simulink model "DiskBrakeThermal"  (R2025b)
settings: Solver=ode45  StartTime=0.0  StopTime=520  MaxStep=0.1  RelTol=1e-6
PreLoadFcn:
  | disk_brake_thermal_params
values from neighbouring files (symbols this model uses):
  A_backing = 0.004    [disk_brake_thermal_params.m]
  A_contact = 0.004    [disk_brake_thermal_params.m]
  A_piston = 0.0012    [disk_brake_thermal_params.m]
  A_rotor = 0.12    [disk_brake_thermal_params.m]
  c_b = 490    [disk_brake_thermal_params.m]
  c_p = 935    [disk_brake_thermal_params.m]
  c_r = 449    [disk_brake_thermal_params.m]
  Cd_A = 0.72    [disk_brake_thermal_params.m]
  Cr = 0.012    [disk_brake_thermal_params.m]
  D = 0.28    [disk_brake_thermal_params.m]
  eps_r = 0.40    (= 0.4)    [disk_brake_thermal_params.m]
  F_drive_max = 7000    [disk_brake_thermal_params.m]
  g = 9.81    [disk_brake_thermal_params.m]
  gamma = 0.95    [disk_brake_thermal_params.m]
  h_nat = 8    [disk_brake_thermal_params.m]
  k_air = 0.026    [disk_brake_thermal_params.m]
  k_cond_pb = k_b * A_backing / t_b    (= 36)    [disk_brake_thermal_params.m]
  k_cond_rp = k_p * A_contact / t_pad    (= 2.9)    [disk_brake_thermal_params.m]
  m_b = 0.25    [disk_brake_thermal_params.m]
  m_p = 0.30    (= 0.3)    [disk_brake_thermal_params.m]
  m_r = 6.0    (= 6)    [disk_brake_thermal_params.m]
  m_veh = 1700    [disk_brake_thermal_params.m]
  mu_air = 1.8e-5    (= 1.8e-05)    [disk_brake_thermal_params.m]
  mu_pad = 0.40    (= 0.4)    [disk_brake_thermal_params.m]
  P_line_max = 120e5    (= 12000000)    [disk_brake_thermal_params.m]
  R_eff = 0.11    [disk_brake_thermal_params.m]
  R_wheel = 0.32    [disk_brake_thermal_params.m]
  rho_air = 1.17    [disk_brake_thermal_params.m]
  rho_air_drag = 1.225    [disk_brake_thermal_params.m]
  sigma = 5.67e-8    (= 5.67e-08)    [disk_brake_thermal_params.m]
  T_amb_init = 25    [disk_brake_thermal_params.m]
  v0 = 27.8    [disk_brake_thermal_params.m]
settings Model: Creator=grouleau  LastModifiedBy=grouleau
settings DataIOCC: ExternalInput=ext_input  LoadExternalInput=on

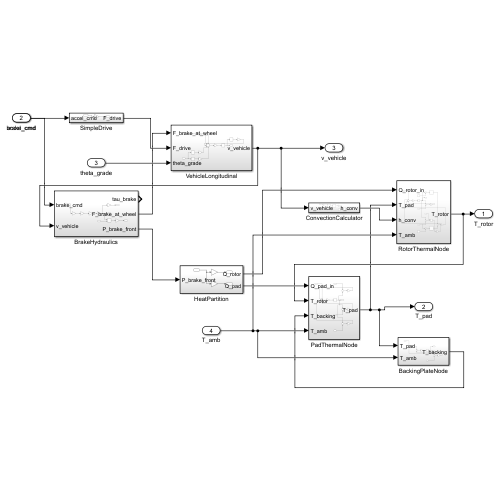
[thumbnail: Simulink's stored preview of the top-level diagram]
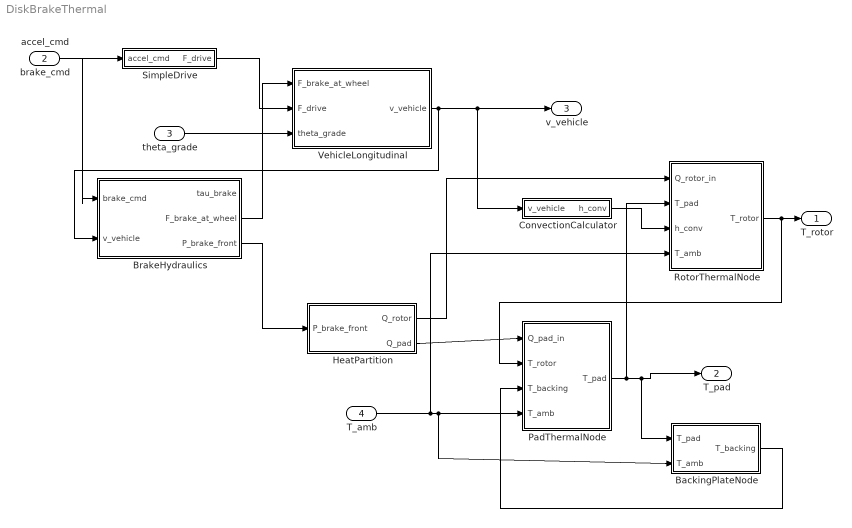
== system DiskBrakeThermal ==
  brake_cmd : Inport
  accel_cmd : Inport  Port=2
  theta_grade : Inport  Port=3
  T_amb : Inport  Port=4
  BackingPlateNode : Subsystem
  BrakeHydraulics : Subsystem
  ConvectionCalculator : Subsystem
  HeatPartition : Subsystem
  PadThermalNode : Subsystem
  RotorThermalNode : Subsystem
  SimpleDrive : Subsystem
  VehicleLongitudinal : Subsystem
  T_rotor : Outport
  T_pad : Outport  Port=2
  v_vehicle : Outport  Port=3
  wires:
  brake_cmd/1 -> BrakeHydraulics/1(brake_cmd)
  accel_cmd/1 -> SimpleDrive/1(accel_cmd)
  theta_grade/1 -> VehicleLongitudinal/3(theta_grade)
  BrakeHydraulics/2(F_brake_at_wheel) -> VehicleLongitudinal/1(F_brake_at_wheel)
  SimpleDrive/1(F_drive) -> VehicleLongitudinal/2(F_drive)
  VehicleLongitudinal/1(v_vehicle) -> v_vehicle/1, ConvectionCalculator/1(v_vehicle), BrakeHydraulics/2(v_vehicle)
  BrakeHydraulics/3(P_brake_front) -> HeatPartition/1(P_brake_front)
  HeatPartition/1(Q_rotor) -> RotorThermalNode/1(Q_rotor_in)
  HeatPartition/2(Q_pad) -> PadThermalNode/1(Q_pad_in)
  ConvectionCalculator/1(h_conv) -> RotorThermalNode/3(h_conv)
  T_amb/1 -> BackingPlateNode/2(T_amb), PadThermalNode/4(T_amb), RotorThermalNode/4(T_amb)
  RotorThermalNode/1(T_rotor) -> PadThermalNode/2(T_rotor), T_rotor/1
  PadThermalNode/1(T_pad) -> T_pad/1, BackingPlateNode/1(T_pad), RotorThermalNode/2(T_pad)
  BackingPlateNode/1(T_backing) -> PadThermalNode/3(T_backing)

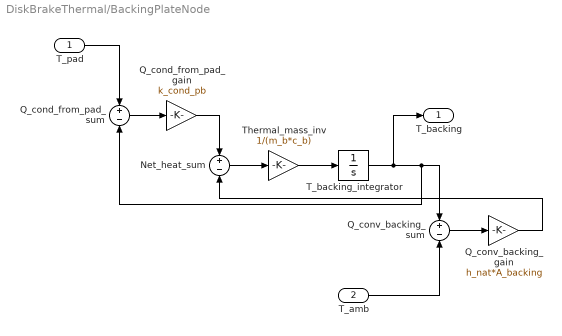
== system DiskBrakeThermal/BackingPlateNode ==
  T_pad : Inport
  T_amb : Inport  Port=2
  Net_heat_sum : Sum  Inputs=+-
  Q_cond_from_pad_gain : Gain  Gain=k_cond_pb
  Q_cond_from_pad_sum : Sum  Inputs=+-
  Q_conv_backing_gain : Gain  Gain=h_nat*A_backing
  Q_conv_backing_sum : Sum  Inputs=+-
  T_backing_integrator : Integrator  InitialCondition=T_amb_init
  Thermal_mass_inv : Gain  Gain=1/(m_b*c_b)
  T_backing : Outport
  wires:
  T_pad/1 -> Q_cond_from_pad_sum/1
  Q_cond_from_pad_sum/1 -> Q_cond_from_pad_gain/1
  Q_conv_backing_sum/1 -> Q_conv_backing_gain/1
  Q_cond_from_pad_gain/1 -> Net_heat_sum/1
  Q_conv_backing_gain/1 -> Net_heat_sum/2
  Net_heat_sum/1 -> Thermal_mass_inv/1
  Thermal_mass_inv/1 -> T_backing_integrator/1
  T_backing_integrator/1 -> Q_conv_backing_sum/1, Q_cond_from_pad_sum/2, T_backing/1
  T_amb/1 -> Q_conv_backing_sum/2

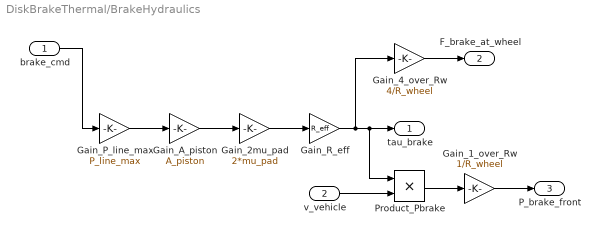
== system DiskBrakeThermal/BrakeHydraulics ==
  brake_cmd : Inport
  v_vehicle : Inport  Port=2
  Gain_1_over_Rw : Gain  Gain=1/R_wheel
  Gain_2mu_pad : Gain  Gain=2*mu_pad
  Gain_4_over_Rw : Gain  Gain=4/R_wheel
  Gain_A_piston : Gain  Gain=A_piston
  Gain_P_line_max : Gain  Gain=P_line_max
  Gain_R_eff : Gain  Gain=R_eff
  Product_Pbrake : Product
  tau_brake : Outport
  F_brake_at_wheel : Outport  Port=2
  P_brake_front : Outport  Port=3
  wires:
  brake_cmd/1 -> Gain_P_line_max/1
  Gain_P_line_max/1 -> Gain_A_piston/1
  Gain_A_piston/1 -> Gain_2mu_pad/1
  Gain_2mu_pad/1 -> Gain_R_eff/1
  Gain_R_eff/1 -> Product_Pbrake/1, tau_brake/1, Gain_4_over_Rw/1
  Gain_4_over_Rw/1 -> F_brake_at_wheel/1
  v_vehicle/1 -> Product_Pbrake/2
  Product_Pbrake/1 -> Gain_1_over_Rw/1
  Gain_1_over_Rw/1 -> P_brake_front/1

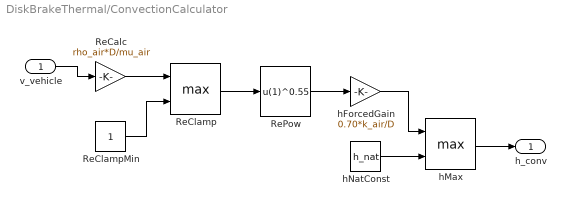
== system DiskBrakeThermal/ConvectionCalculator ==
  v_vehicle : Inport
  ReCalc : Gain  Gain=rho_air*D/mu_air
  ReClamp : MinMax  Function=max  Inputs=2
  ReClampMin : Constant
  RePow : Fcn  Expr=u(1)^0.55
  hForcedGain : Gain  Gain=0.70*k_air/D
  hMax : MinMax  Function=max  Inputs=2
  hNatConst : Constant  Value=h_nat
  h_conv : Outport
  wires:
  v_vehicle/1 -> ReCalc/1
  ReCalc/1 -> ReClamp/1
  ReClampMin/1 -> ReClamp/2
  ReClamp/1 -> RePow/1
  RePow/1 -> hForcedGain/1
  hForcedGain/1 -> hMax/1
  hNatConst/1 -> hMax/2
  hMax/1 -> h_conv/1

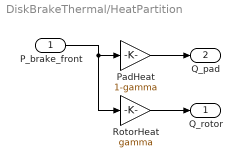
== system DiskBrakeThermal/HeatPartition ==
  P_brake_front : Inport
  PadHeat : Gain  Gain=1-gamma
  RotorHeat : Gain  Gain=gamma
  Q_rotor : Outport
  Q_pad : Outport  Port=2
  wires:
  P_brake_front/1 -> PadHeat/1, RotorHeat/1
  RotorHeat/1 -> Q_rotor/1
  PadHeat/1 -> Q_pad/1

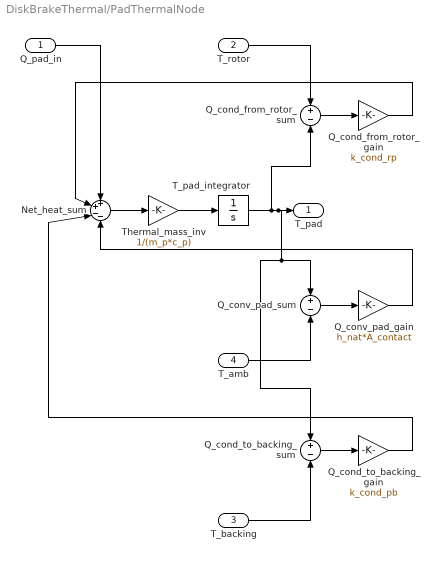
== system DiskBrakeThermal/PadThermalNode ==
  Q_pad_in : Inport
  T_rotor : Inport  Port=2
  T_backing : Inport  Port=3
  T_amb : Inport  Port=4
  Net_heat_sum : Sum  Inputs=++--
  Q_cond_from_rotor_gain : Gain  Gain=k_cond_rp
  Q_cond_from_rotor_sum : Sum  Inputs=+-
  Q_cond_to_backing_gain : Gain  Gain=k_cond_pb
  Q_cond_to_backing_sum : Sum  Inputs=+-
  Q_conv_pad_gain : Gain  Gain=h_nat*A_contact
  Q_conv_pad_sum : Sum  Inputs=+-
  T_pad_integrator : Integrator  InitialCondition=T_amb_init
  Thermal_mass_inv : Gain  Gain=1/(m_p*c_p)
  T_pad : Outport
  wires:
  T_rotor/1 -> Q_cond_from_rotor_sum/1
  Q_cond_from_rotor_sum/1 -> Q_cond_from_rotor_gain/1
  Q_cond_to_backing_sum/1 -> Q_cond_to_backing_gain/1
  Q_conv_pad_sum/1 -> Q_conv_pad_gain/1
  Q_pad_in/1 -> Net_heat_sum/1
  Q_cond_from_rotor_gain/1 -> Net_heat_sum/2
  Q_cond_to_backing_gain/1 -> Net_heat_sum/3
  Q_conv_pad_gain/1 -> Net_heat_sum/4
  Net_heat_sum/1 -> Thermal_mass_inv/1
  Thermal_mass_inv/1 -> T_pad_integrator/1
  T_pad_integrator/1 -> Q_conv_pad_sum/1, Q_cond_to_backing_sum/1, T_pad/1, Q_cond_from_rotor_sum/2
  T_backing/1 -> Q_cond_to_backing_sum/2
  T_amb/1 -> Q_conv_pad_sum/2

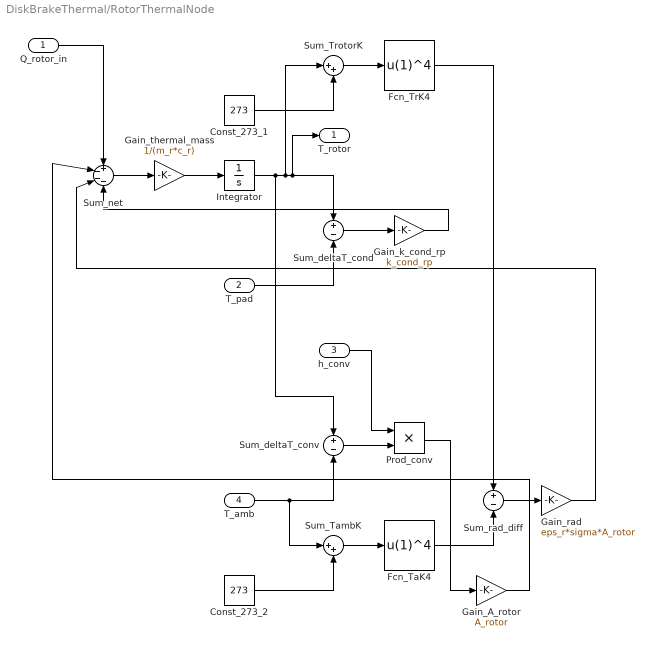
== system DiskBrakeThermal/RotorThermalNode ==
  Q_rotor_in : Inport
  T_pad : Inport  Port=2
  h_conv : Inport  Port=3
  T_amb : Inport  Port=4
  Const_273_1 : Constant  Value=273
  Const_273_2 : Constant  Value=273
  Fcn_TaK4 : Fcn  Expr=u(1)^4
  Fcn_TrK4 : Fcn  Expr=u(1)^4
  Gain_A_rotor : Gain  Gain=A_rotor
  Gain_k_cond_rp : Gain  Gain=k_cond_rp
  Gain_rad : Gain  Gain=eps_r*sigma*A_rotor
  Gain_thermal_mass : Gain  Gain=1/(m_r*c_r)
  Integrator : Integrator  InitialCondition=T_amb_init
  Prod_conv : Product
  Sum_TambK : Sum  Inputs=|++
  Sum_TrotorK : Sum  Inputs=|++
  Sum_deltaT_cond : Sum  Inputs=+-
  Sum_deltaT_conv : Sum  Inputs=+-
  Sum_net : Sum  Inputs=+---
  Sum_rad_diff : Sum  Inputs=+-
  T_rotor : Outport
  wires:
  Integrator/1 -> T_rotor/1, Sum_deltaT_cond/1, Sum_TrotorK/1, Sum_deltaT_conv/1
  T_amb/1 -> Sum_TambK/1, Sum_deltaT_conv/2
  h_conv/1 -> Prod_conv/1
  Sum_deltaT_conv/1 -> Prod_conv/2
  Prod_conv/1 -> Gain_A_rotor/1
  Const_273_1/1 -> Sum_TrotorK/2
  Const_273_2/1 -> Sum_TambK/2
  Sum_TrotorK/1 -> Fcn_TrK4/1
  Sum_TambK/1 -> Fcn_TaK4/1
  Fcn_TrK4/1 -> Sum_rad_diff/1
  Fcn_TaK4/1 -> Sum_rad_diff/2
  Sum_rad_diff/1 -> Gain_rad/1
  T_pad/1 -> Sum_deltaT_cond/2
  Sum_deltaT_cond/1 -> Gain_k_cond_rp/1
  Sum_net/1 -> Gain_thermal_mass/1
  Gain_thermal_mass/1 -> Integrator/1
  Q_rotor_in/1 -> Sum_net/1
  Gain_A_rotor/1 -> Sum_net/2
  Gain_rad/1 -> Sum_net/3
  Gain_k_cond_rp/1 -> Sum_net/4

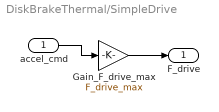
== system DiskBrakeThermal/SimpleDrive ==
  accel_cmd : Inport
  Gain_F_drive_max : Gain  Gain=F_drive_max
  F_drive : Outport
  wires:
  accel_cmd/1 -> Gain_F_drive_max/1
  Gain_F_drive_max/1 -> F_drive/1

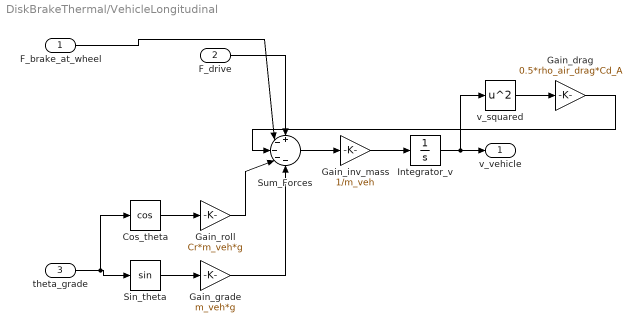
== system DiskBrakeThermal/VehicleLongitudinal ==
  F_brake_at_wheel : Inport
  F_drive : Inport  Port=2
  theta_grade : Inport  Port=3
  Cos_theta : Trigonometry  Operator=cos  ApproximationMethod=CORDIC
  Gain_drag : Gain  Gain=0.5*rho_air_drag*Cd_A
  Gain_grade : Gain  Gain=m_veh*g
  Gain_inv_mass : Gain  Gain=1/m_veh
  Gain_roll : Gain  Gain=Cr*m_veh*g
  Integrator_v : Integrator  InitialCondition=v0  LimitOutput=on  LowerSaturationLimit=0
  Sin_theta : Trigonometry  ApproximationMethod=CORDIC
  Sum_Forces : Sum  Inputs=+----
  v_squared : Math  Operator=square  SignedPower=on  RndMeth=Zero
  v_vehicle : Outport
  wires:
  F_drive/1 -> Sum_Forces/1
  F_brake_at_wheel/1 -> Sum_Forces/2
  Sum_Forces/1 -> Gain_inv_mass/1
  Gain_inv_mass/1 -> Integrator_v/1
  Integrator_v/1 -> v_squared/1, v_vehicle/1
  v_squared/1 -> Gain_drag/1
  theta_grade/1 -> Sin_theta/1, Cos_theta/1
  Cos_theta/1 -> Gain_roll/1
  Sin_theta/1 -> Gain_grade/1
  Gain_drag/1 -> Sum_Forces/3
  Gain_roll/1 -> Sum_Forces/4
  Gain_grade/1 -> Sum_Forces/5
